simulink model "WK3_Problem4"  (R2023a)
settings: Solver=FixedStepAuto  StartTime=0.0  StopTime=30  FixedStep=0.01  RelTol=1e-3
settings Model: Creator=natha  LastModifiedBy=natha

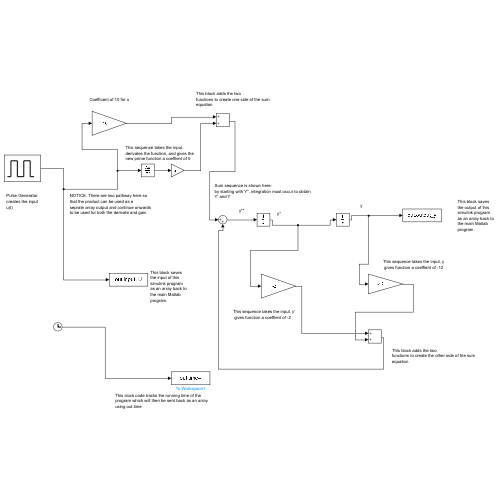
[thumbnail: Simulink's stored preview of the top-level diagram]
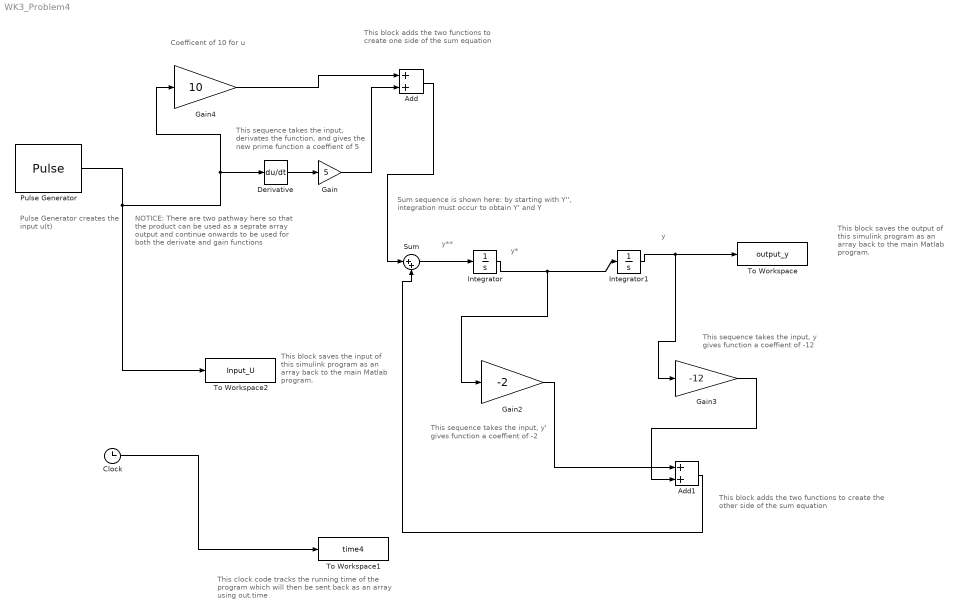
== system WK3_Problem4 ==
  note: Pulse Generator
      | creates the input
      | u(t)
  note: Sum sequence is shown here:
      | by starting with Y'', integration must occur to obtain
      | Y' and Y
  note: Coefficent of 10 for u
  note: This sequence takes the input,
      | derivates the function, and gives the
      | new prime function a coeffient of 5
  note: y
  note: y*
  note: y**
  note: This clock code tracks the running time of the
      | program which will then be sent back as an array
      | using out.time
  note: This block saves
      | the input of this
      | simulink program
      | as an array back to
      | the main Matlab
      | program.
  note: NOTICE: There are two pathway here so
      | that the product can be used as a
      | seprate array output and continue onwards
      | to be used for both the derivate and gain functions
  note: This block adds the two
      | functions to create one side of the sum
      | equation
  note: This sequence takes the input, y'
      |  gives function a coeffient of -2
  note: This sequence takes the input, y
      |  gives function a coeffient of -12
  note: This block adds the two
      | functions to create the other side of the sum
      | equation
  note: This block saves
      | the output of this
      | simulink program
      | as an array back to
      | the main Matlab
      | program.
  Add : Sum
  Add1 : Sum
  Clock : Clock
      settings: Decimation=20
  Derivative : Derivative  CoefficientInTFapproximation=10
  Gain : Gain  Gain=5
  Gain2 : Gain  Gain=-2
  Gain3 : Gain  Gain=-12
  Gain4 : Gain  Gain=10
  Integrator : Integrator
  Integrator1 : Integrator
  Pulse Generator : DiscretePulseGenerator  PulseType=Time based  Amplitude=10  Period=20  PulseWidth=50
  Sum : Sum  Inputs=|++
  To Workspace : ToWorkspace  VariableName=output_y  SampleTime=-1
  To Workspace1 : ToWorkspace  VariableName=time4  SampleTime=-1
  To Workspace2 : ToWorkspace  VariableName=Input_U  SampleTime=-1
  wires:
  Clock/1 -> To Workspace1/1
  Sum/1 -> Integrator/1
  Integrator1/1 -> Gain3/1, To Workspace/1
  Integrator/1 -> Gain2/1, Integrator1/1
  Gain3/1 -> Add1/2
  Add1/1 -> Sum/2
  Gain2/1 -> Add1/1
  Pulse Generator/1 -> To Workspace2/1, Gain4/1, Derivative/1
  Gain4/1 -> Add/1
  Derivative/1 -> Gain/1
  Gain/1 -> Add/2
  Add/1 -> Sum/1
